simulink model "stereo_ibvs_core_backup_20260724_004703"  (R2025b)
settings: Solver=FixedStepDiscrete  StartTime=0.0  StopTime=inf  FixedStep=cfg.Ts  RelTol=1e-3
InitFcn:
  | cfgValid__=evalin('base','exist(''cfg'',''var'')==1 && isstruct(cfg) && all(isfield(cfg,{''Ts'',''robot'',''qInitial'',''zoomInitialSteps'',''cameraIntrinsicsStage1'',''rhoD'',''stereoBaseline'',''centerDesired'',''Kc'',''lambdaC'',''qMin'',''qMax'',''qLimitSoftMargin'',''qDotAlgorithmMax'',''stage1CalibrationReady''}))');if ~cfgValid__,modelFile__=get_param(bdroot,'FileName');modelDir__=fileparts(modelFile__);config1__=fullfile(modelDir__,'stereo_ibvs_config.m');config2__=fullfile(fileparts(modelDir__),'config','stereo_ibvs_config.m');if isfile(config1__),run(config1__);elseif isfile(config2__),run(config2__);else,error('StereoIBVS:ConfigNotFound','找不到stereo_ibvs_config.m。');end;end;clear cfgValid__ modelFile__ modelDir__ config1__ config2__
undefined symbols (not defined in the file): cfg, cfg_baseline, cfg_ekfCovarianceJitter, cfg_ekfInitializationMode, cfg_ekfP0, cfg_ekfRequireNewMeasurement, cfg_ekfSConditionMin, cfg_ekfX0, cfg_focalLength0Mm, cfg_fr3Axis, cfg_fr3Joint8OriginRPY, cfg_fr3Joint8OriginXYZ, cfg_fr3OriginRPY, cfg_fr3OriginXYZ, cfg_numericalEpsilon, cfg_pixelNoiseStd, cfg_q0, cfg_rhoMax, cfg_rhoMin, cfg_sigmaJerk, cfg_T_CL_CR, cfg_T_link8_CL, cfg_T_W_B, cfg_Ts, cfg_visibilityZMin
(part 2 of 4)

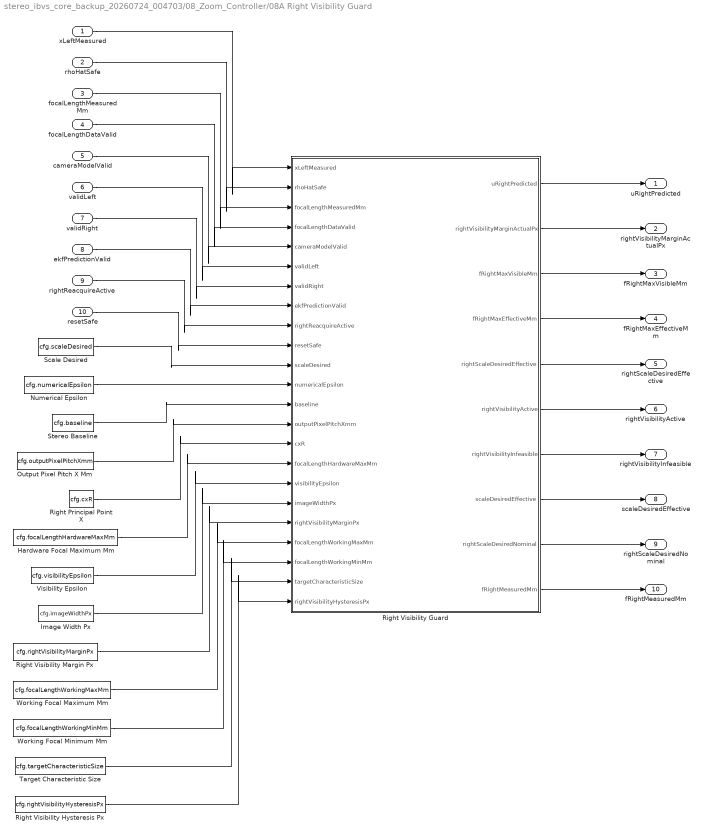
== system stereo_ibvs_core_backup_20260724_004703/08_Zoom_Controller/08A Right Visibility Guard ==
  xLeftMeasured : Inport  OutDataTypeStr=double  PortDimensions=1
  rhoHatSafe : Inport  Port=2  OutDataTypeStr=double  PortDimensions=1
  focalLengthMeasuredMm : Inport  Port=3  OutDataTypeStr=double  PortDimensions=[2 1]
  focalLengthDataValid : Inport  Port=4  OutDataTypeStr=double  PortDimensions=1
  cameraModelValid : Inport  Port=5  OutDataTypeStr=double  PortDimensions=1
  validLeft : Inport  Port=6  OutDataTypeStr=double  PortDimensions=1
  validRight : Inport  Port=7  OutDataTypeStr=double  PortDimensions=1
  ekfPredictionValid : Inport  Port=8  OutDataTypeStr=double  PortDimensions=1
  rightReacquireActive : Inport  Port=9  OutDataTypeStr=double  PortDimensions=1
  resetSafe : Inport  Port=10  OutDataTypeStr=double  PortDimensions=1
  Hardware Focal Maximum Mm : Constant  Value=cfg.focalLengthHardwareMaxMm  OutDataTypeStr=double  SampleTime=-1
  Image Width Px : Constant  Value=cfg.imageWidthPx  OutDataTypeStr=double  SampleTime=-1
  Numerical Epsilon : Constant  Value=cfg.numericalEpsilon  OutDataTypeStr=double  SampleTime=-1
  Output Pixel Pitch X Mm : Constant  Value=cfg.outputPixelPitchXmm  OutDataTypeStr=double  SampleTime=-1
  Right Principal Point X : Constant  Value=cfg.cxR  OutDataTypeStr=double  SampleTime=-1
  Right Visibility Guard : MATLAB Function  TreatAsAtomicUnit=on
  Right Visibility Hysteresis Px : Constant  Value=cfg.rightVisibilityHysteresisPx  OutDataTypeStr=double  SampleTime=-1
  Right Visibility Margin Px : Constant  Value=cfg.rightVisibilityMarginPx  OutDataTypeStr=double  SampleTime=-1
  Scale Desired : Constant  Value=cfg.scaleDesired  OutDataTypeStr=double  SampleTime=-1
  Stereo Baseline : Constant  Value=cfg.baseline  OutDataTypeStr=double  SampleTime=-1
  Target Characteristic Size : Constant  Value=cfg.targetCharacteristicSize  OutDataTypeStr=double  SampleTime=-1
  Visibility Epsilon : Constant  Value=cfg.visibilityEpsilon  OutDataTypeStr=double  SampleTime=-1
  Working Focal Maximum Mm : Constant  Value=cfg.focalLengthWorkingMaxMm  OutDataTypeStr=double  SampleTime=-1
  Working Focal Minimum Mm : Constant  Value=cfg.focalLengthWorkingMinMm  OutDataTypeStr=double  SampleTime=-1
  uRightPredicted : Outport  PortDimensions=1
  rightVisibilityMarginActualPx : Outport  Port=2  PortDimensions=1
  fRightMaxVisibleMm : Outport  Port=3  PortDimensions=1
  fRightMaxEffectiveMm : Outport  Port=4  PortDimensions=1
  rightScaleDesiredEffective : Outport  Port=5  PortDimensions=1
  rightVisibilityActive : Outport  Port=6  PortDimensions=1
  rightVisibilityInfeasible : Outport  Port=7  PortDimensions=1
  scaleDesiredEffective : Outport  Port=8  PortDimensions=[2 1]
  rightScaleDesiredNominal : Outport  Port=9  PortDimensions=1
  fRightMeasuredMm : Outport  Port=10  PortDimensions=1
  wires:
  Right Visibility Guard/9(rightScaleDesiredNominal) -> rightScaleDesiredNominal/1
  Right Visibility Guard/7(rightVisibilityInfeasible) -> rightVisibilityInfeasible/1
  Scale Desired/1 -> Right Visibility Guard/11(scaleDesired)
  Right Visibility Guard/6(rightVisibilityActive) -> rightVisibilityActive/1
  rightReacquireActive/1 -> Right Visibility Guard/9(rightReacquireActive)
  ekfPredictionValid/1 -> Right Visibility Guard/8(ekfPredictionValid)
  resetSafe/1 -> Right Visibility Guard/10(resetSafe)
  Stereo Baseline/1 -> Right Visibility Guard/13(baseline)
  validLeft/1 -> Right Visibility Guard/6(validLeft)
  Working Focal Minimum Mm/1 -> Right Visibility Guard/21(focalLengthWorkingMinMm)
  rhoHatSafe/1 -> Right Visibility Guard/2(rhoHatSafe)
  focalLengthDataValid/1 -> Right Visibility Guard/4(focalLengthDataValid)
  cameraModelValid/1 -> Right Visibility Guard/5(cameraModelValid)
  validRight/1 -> Right Visibility Guard/7(validRight)
  Right Visibility Guard/8(scaleDesiredEffective) -> scaleDesiredEffective/1
  Hardware Focal Maximum Mm/1 -> Right Visibility Guard/16(focalLengthHardwareMaxMm)
  Image Width Px/1 -> Right Visibility Guard/18(imageWidthPx)
  Output Pixel Pitch X Mm/1 -> Right Visibility Guard/14(outputPixelPitchXmm)
  Right Visibility Guard/10(fRightMeasuredMm) -> fRightMeasuredMm/1
  Right Principal Point X/1 -> Right Visibility Guard/15(cxR)
  Target Characteristic Size/1 -> Right Visibility Guard/22(targetCharacteristicSize)
  Visibility Epsilon/1 -> Right Visibility Guard/17(visibilityEpsilon)
  Right Visibility Guard/2(rightVisibilityMarginActualPx) -> rightVisibilityMarginActualPx/1
  Right Visibility Guard/4(fRightMaxEffectiveMm) -> fRightMaxEffectiveMm/1
  Numerical Epsilon/1 -> Right Visibility Guard/12(numericalEpsilon)
  Right Visibility Guard/3(fRightMaxVisibleMm) -> fRightMaxVisibleMm/1
  Working Focal Maximum Mm/1 -> Right Visibility Guard/20(focalLengthWorkingMaxMm)
  Right Visibility Guard/1(uRightPredicted) -> uRightPredicted/1
  Right Visibility Margin Px/1 -> Right Visibility Guard/19(rightVisibilityMarginPx)
  Right Visibility Hysteresis Px/1 -> Right Visibility Guard/23(rightVisibilityHysteresisPx)
  focalLengthMeasuredMm/1 -> Right Visibility Guard/3(focalLengthMeasuredMm)
  xLeftMeasured/1 -> Right Visibility Guard/1(xLeftMeasured)
  Right Visibility Guard/5(rightScaleDesiredEffective) -> rightScaleDesiredEffective/1

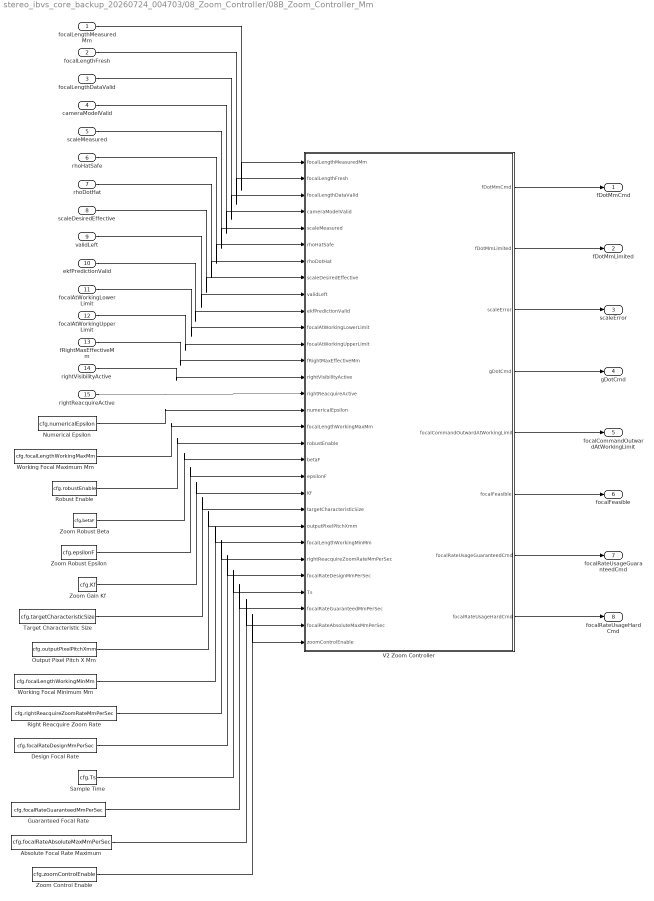
== system stereo_ibvs_core_backup_20260724_004703/08_Zoom_Controller/08B_Zoom_Controller_Mm ==
  focalLengthMeasuredMm : Inport  OutDataTypeStr=double  PortDimensions=[2 1]
  focalLengthFresh : Inport  Port=2  OutDataTypeStr=double  PortDimensions=1
  focalLengthDataValid : Inport  Port=3  OutDataTypeStr=double  PortDimensions=1
  cameraModelValid : Inport  Port=4  OutDataTypeStr=double  PortDimensions=1
  scaleMeasured : Inport  Port=5  OutDataTypeStr=double  PortDimensions=[2 1]
  rhoHatSafe : Inport  Port=6  OutDataTypeStr=double  PortDimensions=1
  rhoDotHat : Inport  Port=7  OutDataTypeStr=double  PortDimensions=[2 1]
  scaleDesiredEffective : Inport  Port=8  OutDataTypeStr=double  PortDimensions=[2 1]
  validLeft : Inport  Port=9  OutDataTypeStr=double  PortDimensions=1
  ekfPredictionValid : Inport  Port=10  OutDataTypeStr=double  PortDimensions=1
  focalAtWorkingLowerLimit : Inport  Port=11  OutDataTypeStr=double  PortDimensions=[2 1]
  focalAtWorkingUpperLimit : Inport  Port=12  OutDataTypeStr=double  PortDimensions=[2 1]
  fRightMaxEffectiveMm : Inport  Port=13  OutDataTypeStr=double  PortDimensions=1
  rightVisibilityActive : Inport  Port=14  OutDataTypeStr=double  PortDimensions=1
  rightReacquireActive : Inport  Port=15  OutDataTypeStr=double  PortDimensions=1
  Absolute Focal Rate Maximum : Constant  Value=cfg.focalRateAbsoluteMaxMmPerSec  OutDataTypeStr=double  SampleTime=-1
  Design Focal Rate : Constant  Value=cfg.focalRateDesignMmPerSec  OutDataTypeStr=double  SampleTime=-1
  Guaranteed Focal Rate : Constant  Value=cfg.focalRateGuaranteedMmPerSec  OutDataTypeStr=double  SampleTime=-1
  Numerical Epsilon : Constant  Value=cfg.numericalEpsilon  OutDataTypeStr=double  SampleTime=-1
  Output Pixel Pitch X Mm : Constant  Value=cfg.outputPixelPitchXmm  OutDataTypeStr=double  SampleTime=-1
  Right Reacquire Zoom Rate : Constant  Value=cfg.rightReacquireZoomRateMmPerSec  OutDataTypeStr=double  SampleTime=-1
  Robust Enable : Constant  Value=cfg.robustEnable  OutDataTypeStr=double  SampleTime=-1
  Sample Time : Constant  Value=cfg.Ts  OutDataTypeStr=double  SampleTime=-1
  Target Characteristic Size : Constant  Value=cfg.targetCharacteristicSize  OutDataTypeStr=double  SampleTime=-1
  V2 Zoom Controller : MATLAB Function  TreatAsAtomicUnit=on
  Working Focal Maximum Mm : Constant  Value=cfg.focalLengthWorkingMaxMm  OutDataTypeStr=double  SampleTime=-1
  Working Focal Minimum Mm : Constant  Value=cfg.focalLengthWorkingMinMm  OutDataTypeStr=double  SampleTime=-1
  Zoom Control Enable : Constant  Value=cfg.zoomControlEnable  OutDataTypeStr=double  SampleTime=-1
  Zoom Gain Kf : Constant  Value=cfg.Kf  OutDataTypeStr=double  SampleTime=-1
  Zoom Robust Beta : Constant  Value=cfg.betaF  OutDataTypeStr=double  SampleTime=-1
  Zoom Robust Epsilon : Constant  Value=cfg.epsilonF  OutDataTypeStr=double  SampleTime=-1
  fDotMmCmd : Outport  PortDimensions=[2 1]
  fDotMmLimited : Outport  Port=2  PortDimensions=[2 1]
  scaleError : Outport  Port=3  PortDimensions=[2 1]
  gDotCmd : Outport  Port=4  PortDimensions=[2 1]
  focalCommandOutwardAtWorkingLimit : Outport  Port=5  PortDimensions=[2 1]
  focalFeasible : Outport  Port=6  PortDimensions=[2 1]
  focalRateUsageGuaranteedCmd : Outport  Port=7  PortDimensions=[2 1]
  focalRateUsageHardCmd : Outport  Port=8  PortDimensions=[2 1]
  wires:
  V2 Zoom Controller/6(focalFeasible) -> focalFeasible/1
  V2 Zoom Controller/4(gDotCmd) -> gDotCmd/1
  V2 Zoom Controller/3(scaleError) -> scaleError/1
  V2 Zoom Controller/1(fDotMmCmd) -> fDotMmCmd/1
  Zoom Control Enable/1 -> V2 Zoom Controller/30(zoomControlEnable)
  V2 Zoom Controller/8(focalRateUsageHardCmd) -> focalRateUsageHardCmd/1
  focalAtWorkingUpperLimit/1 -> V2 Zoom Controller/12(focalAtWorkingUpperLimit)
  ekfPredictionValid/1 -> V2 Zoom Controller/10(ekfPredictionValid)
  V2 Zoom Controller/5(focalCommandOutwardAtWorkingLimit) -> focalCommandOutwardAtWorkingLimit/1
  focalAtWorkingLowerLimit/1 -> V2 Zoom Controller/11(focalAtWorkingLowerLimit)
  Zoom Gain Kf/1 -> V2 Zoom Controller/21(Kf)
  scaleMeasured/1 -> V2 Zoom Controller/5(scaleMeasured)
  rhoDotHat/1 -> V2 Zoom Controller/7(rhoDotHat)
  rhoHatSafe/1 -> V2 Zoom Controller/6(rhoHatSafe)
  V2 Zoom Controller/2(fDotMmLimited) -> fDotMmLimited/1
  Working Focal Maximum Mm/1 -> V2 Zoom Controller/17(focalLengthWorkingMaxMm)
  focalLengthDataValid/1 -> V2 Zoom Controller/3(focalLengthDataValid)
  focalLengthFresh/1 -> V2 Zoom Controller/2(focalLengthFresh)
  fRightMaxEffectiveMm/1 -> V2 Zoom Controller/13(fRightMaxEffectiveMm)
  validLeft/1 -> V2 Zoom Controller/9(validLeft)
  Numerical Epsilon/1 -> V2 Zoom Controller/16(numericalEpsilon)
  focalLengthMeasuredMm/1 -> V2 Zoom Controller/1(focalLengthMeasuredMm)
  Working Focal Minimum Mm/1 -> V2 Zoom Controller/24(focalLengthWorkingMinMm)
  rightReacquireActive/1 -> V2 Zoom Controller/15(rightReacquireActive)
  Robust Enable/1 -> V2 Zoom Controller/18(robustEnable)
  Target Characteristic Size/1 -> V2 Zoom Controller/22(targetCharacteristicSize)
  rightVisibilityActive/1 -> V2 Zoom Controller/14(rightVisibilityActive)
  cameraModelValid/1 -> V2 Zoom Controller/4(cameraModelValid)
  Zoom Robust Beta/1 -> V2 Zoom Controller/19(betaF)
  scaleDesiredEffective/1 -> V2 Zoom Controller/8(scaleDesiredEffective)
  Zoom Robust Epsilon/1 -> V2 Zoom Controller/20(epsilonF)
  Output Pixel Pitch X Mm/1 -> V2 Zoom Controller/23(outputPixelPitchXmm)
  Design Focal Rate/1 -> V2 Zoom Controller/26(focalRateDesignMmPerSec)
  Sample Time/1 -> V2 Zoom Controller/27(Ts)
  Guaranteed Focal Rate/1 -> V2 Zoom Controller/28(focalRateGuaranteedMmPerSec)
  V2 Zoom Controller/7(focalRateUsageGuaranteedCmd) -> focalRateUsageGuaranteedCmd/1
  Right Reacquire Zoom Rate/1 -> V2 Zoom Controller/25(rightReacquireZoomRateMmPerSec)
  Absolute Focal Rate Maximum/1 -> V2 Zoom Controller/29(focalRateAbsoluteMaxMmPerSec)

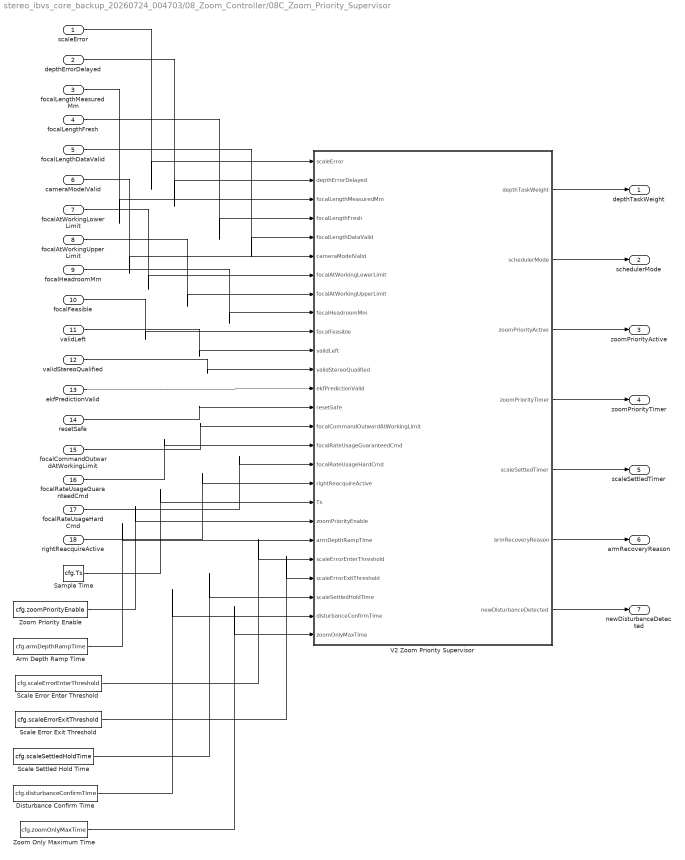
== system stereo_ibvs_core_backup_20260724_004703/08_Zoom_Controller/08C_Zoom_Priority_Supervisor ==
  scaleError : Inport  OutDataTypeStr=double  PortDimensions=[2 1]
  depthErrorDelayed : Inport  Port=2  OutDataTypeStr=double  PortDimensions=1
  focalLengthMeasuredMm : Inport  Port=3  OutDataTypeStr=double  PortDimensions=[2 1]
  focalLengthFresh : Inport  Port=4  OutDataTypeStr=double  PortDimensions=1
  focalLengthDataValid : Inport  Port=5  OutDataTypeStr=double  PortDimensions=1
  cameraModelValid : Inport  Port=6  OutDataTypeStr=double  PortDimensions=1
  focalAtWorkingLowerLimit : Inport  Port=7  OutDataTypeStr=double  PortDimensions=[2 1]
  focalAtWorkingUpperLimit : Inport  Port=8  OutDataTypeStr=double  PortDimensions=[2 1]
  focalHeadroomMm : Inport  Port=9  OutDataTypeStr=double  PortDimensions=[2 1]
  focalFeasible : Inport  Port=10  OutDataTypeStr=double  PortDimensions=[2 1]
  validLeft : Inport  Port=11  OutDataTypeStr=double  PortDimensions=1
  validStereoQualified : Inport  Port=12  OutDataTypeStr=double  PortDimensions=1
  ekfPredictionValid : Inport  Port=13  OutDataTypeStr=double  PortDimensions=1
  resetSafe : Inport  Port=14  OutDataTypeStr=double  PortDimensions=1
  focalCommandOutwardAtWorkingLimit : Inport  Port=15  OutDataTypeStr=double  PortDimensions=[2 1]
  focalRateUsageGuaranteedCmd : Inport  Port=16  OutDataTypeStr=double  PortDimensions=[2 1]
  focalRateUsageHardCmd : Inport  Port=17  OutDataTypeStr=double  PortDimensions=[2 1]
  rightReacquireActive : Inport  Port=18  OutDataTypeStr=double  PortDimensions=1
  Arm Depth Ramp Time : Constant  Value=cfg.armDepthRampTime  OutDataTypeStr=double  SampleTime=-1
  Disturbance Confirm Time : Constant  Value=cfg.disturbanceConfirmTime  OutDataTypeStr=double  SampleTime=-1
  Sample Time : Constant  Value=cfg.Ts  OutDataTypeStr=double  SampleTime=-1
  Scale Error Enter Threshold : Constant  Value=cfg.scaleErrorEnterThreshold  OutDataTypeStr=double  SampleTime=-1
  Scale Error Exit Threshold : Constant  Value=cfg.scaleErrorExitThreshold  OutDataTypeStr=double  SampleTime=-1
  Scale Settled Hold Time : Constant  Value=cfg.scaleSettledHoldTime  OutDataTypeStr=double  SampleTime=-1
  V2 Zoom Priority Supervisor : MATLAB Function  TreatAsAtomicUnit=on
  Zoom Only Maximum Time : Constant  Value=cfg.zoomOnlyMaxTime  OutDataTypeStr=double  SampleTime=-1
  Zoom Priority Enable : Constant  Value=cfg.zoomPriorityEnable  OutDataTypeStr=double  SampleTime=-1
  depthTaskWeight : Outport  PortDimensions=1
  schedulerMode : Outport  Port=2  PortDimensions=1
  zoomPriorityActive : Outport  Port=3  PortDimensions=1
  zoomPriorityTimer : Outport  Port=4  PortDimensions=1
  scaleSettledTimer : Outport  Port=5  PortDimensions=1
  armRecoveryReason : Outport  Port=6  PortDimensions=1
  newDisturbanceDetected : Outport  Port=7  PortDimensions=1
  wires:
  V2 Zoom Priority Supervisor/7(newDisturbanceDetected) -> newDisturbanceDetected/1
  V2 Zoom Priority Supervisor/6(armRecoveryReason) -> armRecoveryReason/1
  V2 Zoom Priority Supervisor/4(zoomPriorityTimer) -> zoomPriorityTimer/1
  validLeft/1 -> V2 Zoom Priority Supervisor/11(validLeft)
  focalFeasible/1 -> V2 Zoom Priority Supervisor/10(focalFeasible)
  ekfPredictionValid/1 -> V2 Zoom Priority Supervisor/13(ekfPredictionValid)
  focalAtWorkingLowerLimit/1 -> V2 Zoom Priority Supervisor/7(focalAtWorkingLowerLimit)
  Zoom Only Maximum Time/1 -> V2 Zoom Priority Supervisor/26(zoomOnlyMaxTime)
  cameraModelValid/1 -> V2 Zoom Priority Supervisor/6(cameraModelValid)
  scaleError/1 -> V2 Zoom Priority Supervisor/1(scaleError)
  focalLengthDataValid/1 -> V2 Zoom Priority Supervisor/5(focalLengthDataValid)
  focalRateUsageHardCmd/1 -> V2 Zoom Priority Supervisor/17(focalRateUsageHardCmd)
  V2 Zoom Priority Supervisor/5(scaleSettledTimer) -> scaleSettledTimer/1
  V2 Zoom Priority Supervisor/2(schedulerMode) -> schedulerMode/1
  focalLengthFresh/1 -> V2 Zoom Priority Supervisor/4(focalLengthFresh)
  Scale Settled Hold Time/1 -> V2 Zoom Priority Supervisor/24(scaleSettledHoldTime)
  V2 Zoom Priority Supervisor/1(depthTaskWeight) -> depthTaskWeight/1
  resetSafe/1 -> V2 Zoom Priority Supervisor/14(resetSafe)
  focalRateUsageGuaranteedCmd/1 -> V2 Zoom Priority Supervisor/16(focalRateUsageGuaranteedCmd)
  rightReacquireActive/1 -> V2 Zoom Priority Supervisor/18(rightReacquireActive)
  Sample Time/1 -> V2 Zoom Priority Supervisor/19(Ts)
  focalAtWorkingUpperLimit/1 -> V2 Zoom Priority Supervisor/8(focalAtWorkingUpperLimit)
  focalCommandOutwardAtWorkingLimit/1 -> V2 Zoom Priority Supervisor/15(focalCommandOutwardAtWorkingLimit)
  Zoom Priority Enable/1 -> V2 Zoom Priority Supervisor/20(zoomPriorityEnable)
  depthErrorDelayed/1 -> V2 Zoom Priority Supervisor/2(depthErrorDelayed)
  Arm Depth Ramp Time/1 -> V2 Zoom Priority Supervisor/21(armDepthRampTime)
  Scale Error Enter Threshold/1 -> V2 Zoom Priority Supervisor/22(scaleErrorEnterThreshold)
  Scale Error Exit Threshold/1 -> V2 Zoom Priority Supervisor/23(scaleErrorExitThreshold)
  validStereoQualified/1 -> V2 Zoom Priority Supervisor/12(validStereoQualified)
  focalHeadroomMm/1 -> V2 Zoom Priority Supervisor/9(focalHeadroomMm)
  Disturbance Confirm Time/1 -> V2 Zoom Priority Supervisor/25(disturbanceConfirmTime)
  focalLengthMeasuredMm/1 -> V2 Zoom Priority Supervisor/3(focalLengthMeasuredMm)
  V2 Zoom Priority Supervisor/3(zoomPriorityActive) -> zoomPriorityActive/1

== matlab function stereo_ibvs_core_backup_20260724_004703/02_Camera_and_Zoom_Model/V2_Camera_and_Zoom_Model ==
  data: focalLengthMeasuredMmRaw input; focalLengthMeasuredMm output; focalLengthIsNew input; resetSafe input; cfg_focalLengthHardwareMinMm input; cfg_focalLengthHardwareMaxMm input; cfg_focalLengthWorkingMinMm input; cfg_focalLengthWorkingMaxMm input; cfg_outputPixelPitchXmm input; cfg_outputPixelPitchYmm input; cfg_focalLengthTimeoutFrames input; cfg_numericalEpsilon input; fxMeasuredPx output; fyMeasuredPx output; focalLengthFresh output; focalLengthDataValid output; focalAtWorkingLowerLimit output; focalAtWorkingUpperLimit output; focalAtHardwareLowerLimit output; focalAtHardwareUpperLimit output; focalOutsideWorkingRange output; focalHardwareLimitViolation output; focalRangeUsage output; focalHeadroomMm output; cameraModelValid output
function [ ...
    focalLengthMeasuredMm, ...
    fxMeasuredPx, ...
    fyMeasuredPx, ...
    focalLengthFresh, ...
    focalLengthDataValid, ...
    focalAtWorkingLowerLimit, ...
    focalAtWorkingUpperLimit, ...
    focalAtHardwareLowerLimit, ...
    focalAtHardwareUpperLimit, ...
    focalOutsideWorkingRange, ...
    focalHardwareLimitViolation, ...
    focalRangeUsage, ...
    focalHeadroomMm, ...
    cameraModelValid] = fcn( ...
    focalLengthMeasuredMmRaw, ...
    focalLengthIsNew, ...
    resetSafe, ...
    cfg_focalLengthHardwareMinMm, ...
    cfg_focalLengthHardwareMaxMm, ...
    cfg_focalLengthWorkingMinMm, ...
    cfg_focalLengthWorkingMaxMm, ...
    cfg_outputPixelPitchXmm, ...
    cfg_outputPixelPitchYmm, ...
    cfg_focalLengthTimeoutFrames, ...
    cfg_numericalEpsilon)
%#codegen
% V2 Camera and Zoom Model
%
% 焦距反馈：
% [fL_mm; fR_mm]
%
% 超时后保持最后一次有效焦距，但 focalLengthFresh = false。
% 08模块应在 focalLengthFresh = false 时停止Zoom命令。

%% 固定尺寸输入
focalRaw = reshape(focalLengthMeasuredMmRaw,2,1);

hardwareMin = reshape( ...
    cfg_focalLengthHardwareMinMm,2,1);

hardwareMax = reshape( ...
    cfg_focalLengthHardwareMaxMm,2,1);

workingMin = reshape( ...
    cfg_focalLengthWorkingMinMm,2,1);

workingMax = reshape( ...
    cfg_focalLengthWorkingMaxMm,2,1);

%% 持久状态
persistent lastValidFocalLengthMm
persistent focalLengthReceivedOnce
persistent framesSinceLastValidMessage

if isempty(lastValidFocalLengthMm)
    lastValidFocalLengthMm = zeros(2,1);
    focalLengthReceivedOnce = false;
    framesSinceLastValidMessage = ...
        double(cfg_focalLengthTimeoutFrames);
end

%% 固定尺寸输出
focalLengthMeasuredMm = zeros(2,1);
fxMeasuredPx = zeros(2,1);
fyMeasuredPx = zeros(2,1);

focalLengthFresh = false;
focalLengthDataValid = false;

focalAtWorkingLowerLimit = false(2,1);
focalAtWorkingUpperLimit = false(2,1);
focalAtHardwareLowerLimit = false(2,1);
focalAtHardwareUpperLimit = false(2,1);

focalOutsideWorkingRange = false(2,1);
focalHardwareLimitViolation = false(2,1);

focalRangeUsage = zeros(2,1);
focalHeadroomMm = zeros(2,1);

cameraModelValid = false;

%% 配置检查
numericalConfigurationValid = ...
    isfinite(cfg_numericalEpsilon) && ...
    cfg_numericalEpsilon > 0;

hardwareRangeValid = ...
    all(isfinite(hardwareMin)) && ...
    all(isfinite(hardwareMax)) && ...
    all(hardwareMax > hardwareMin);

workingRangeValid = ...
    all(isfinite(workingMin)) && ...
    all(isfinite(workingMax)) && ...
    all(workingMax > workingMin) && ...
    all(workingMin >= hardwareMin) && ...
    all(workingMax <= hardwareMax);

pixelPitchValid = ...
    isfinite(cfg_outputPixelPitchXmm) && ...
    isfinite(cfg_outputPixelPitchYmm) && ...
    cfg_outputPixelPitchXmm > cfg_numericalEpsilon && ...
    cfg_outputPixelPitchYmm > cfg_numericalEpsilon;

timeoutConfigurationValid = ...
    isfinite(cfg_focalLengthTimeoutFrames) && ...
    cfg_focalLengthTimeoutFrames >= 1;

configurationValid = ...
    numericalConfigurationValid && ...
    hardwareRangeValid && ...
    workingRangeValid && ...
    pixelPitchValid && ...
    timeoutConfigurationValid;

%% 控制输入检查
controlSignalsFinite = ...
    isfinite(focalLengthIsNew) && ...
    isfinite(resetSafe);

%% 复位或更新焦距状态
if ~controlSignalsFinite || resetSafe > 0.5

    lastValidFocalLengthMm = zeros(2,1);
    focalLengthReceivedOnce = false;
    framesSinceLastValidMessage = ...
        double(cfg_focalLengthTimeoutFrames);

else

    rawFinite = all(isfinite(focalRaw));

    rawInsideHardwareRange = ...
        rawFinite && ...
        hardwareRangeValid && ...
        all(focalRaw >= hardwareMin) && ...
        all(focalRaw <= hardwareMax);

    newValidMessage = ...
        focalLengthIsNew > 0.5 && ...
        rawInsideHardwareRange && ...
        configurationValid;

    if newValidMessage

        lastValidFocalLengthMm = focalRaw;
        focalLengthReceivedOnce = true;
        framesSinceLastValidMessage = 0;

    elseif focalLengthReceivedOnce

        maximumCounterValue = ...
            double(cfg_focalLengthTimeoutFrames) + 1;

        framesSinceLastValidMessage = min( ...
            framesSinceLastValidMessage + 1, ...
            maximumCounterValue);
    end
end

%% 输出最近一次有效焦距
if focalLengthReceivedOnce
    focalLengthMeasuredMm = ...
        lastValidFocalLengthMm;
end

%% 焦距新鲜度
focalLengthFresh = ...
    focalLengthReceivedOnce && ...
    framesSinceLastValidMessage < ...
        double(cfg_focalLengthTimeoutFrames);

%% 保存焦距有效性
if focalLengthReceivedOnce && hardwareRangeValid

    focalLengthDataValid = ...
        all(isfinite(focalLengthMeasuredMm)) && ...
        all(focalLengthMeasuredMm >= hardwareMin) && ...
        all(focalLengthMeasuredMm <= hardwareMax);
end

%% 焦距范围状态
if focalLengthReceivedOnce && configurationValid

    focalAtWorkingLowerLimit = ...
        focalLengthMeasuredMm <= workingMin;

    focalAtWorkingUpperLimit = ...
        focalLengthMeasuredMm >= workingMax;

    focalAtHardwareLowerLimit = ...
        focalLengthMeasuredMm <= hardwareMin;

    focalAtHardwareUpperLimit = ...
        focalLengthMeasuredMm >= hardwareMax;

    focalOutsideWorkingRange = ...
        focalLengthMeasuredMm < workingMin | ...
        focalLengthMeasuredMm > workingMax;

    focalHardwareLimitViolation = ...
        focalLengthMeasuredMm < hardwareMin | ...
        focalLengthMeasuredMm > hardwareMax;

    workingRangeWidth = ...
        workingMax - workingMin;

    focalRangeUsage = ...
        (focalLengthMeasuredMm-workingMin) ./ ...
        workingRangeWidth;

    focalRangeUsage = min( ...
        max(focalRangeUsage,zeros(2,1)), ...
        ones(2,1));

    lowerHeadroomMm = ...
        focalLengthMeasuredMm-workingMin;

    upperHeadroomMm = ...
        workingMax-focalLengthMeasuredMm;

    focalHeadroomMm = max( ...
        min(lowerHeadroomMm,upperHeadroomMm), ...
        zeros(2,1));
end

%% 焦距mm转换为像素焦距
cameraModelValid = ...
    configurationValid && ...
    focalLengthDataValid && ...
    ~any(focalHardwareLimitViolation);

if cameraModelValid

    fxMeasuredPx = ...
        focalLengthMeasuredMm ./ ...
        cfg_outputPixelPitchXmm;

    fyMeasuredPx = ...
        focalLengthMeasuredMm ./ ...
        cfg_outputPixelPitchYmm;
end

%% 最终有限值保护
outputFinite = ...
    all(isfinite(focalLengthMeasuredMm)) && ...
    all(isfinite(fxMeasuredPx)) && ...
    all(isfinite(fyMeasuredPx)) && ...
    all(isfinite(focalRangeUsage)) && ...
    all(isfinite(focalHeadroomMm));

if ~outputFinite

    focalLengthMeasuredMm = zeros(2,1);
    fxMeasuredPx = zeros(2,1);
    fyMeasuredPx = zeros(2,1);

    focalLengthFresh = false;
    focalLengthDataValid = false;

    focalAtWorkingLowerLimit = false(2,1);
    focalAtWorkingUpperLimit = false(2,1);
    focalAtHardwareLowerLimit = false(2,1);
    focalAtHardwareUpperLimit = false(2,1);

    focalOutsideWorkingRange = false(2,1);
    focalHardwareLimitViolation = false(2,1);

    focalRangeUsage = zeros(2,1);
    focalHeadroomMm = zeros(2,1);

    cameraModelValid = false;
end
end

== matlab function stereo_ibvs_core_backup_20260724_004703/07_Arm_Priority_Controller/Final Arm Priority Controller ==
  data: q input; qDotCmd output; cLMeasured input; rhoHatL input; vHatLeft input; JL input; cLd input; rhoD input; validLeft input; ekfPredictionValid input; centerEnable input; depthEnable input; armEnable input; depthTaskWeight input; cfg_numericalEpsilon input; cfg_robustEnable input; cfg_betaC input; cfg_epsilonC input; cfg_Kc input; cfg_lambdaC input; cfg_betaRho input; cfg_epsilonRho input; cfg_kRho input; cfg_lambdaRho input; cfg_nullspaceEnable input; cfg_kNull input; cfg_qMid input; cfg_leftOnlyCenterControlEnable input; centerError output; depthError output; rcondJc output; rcondArho output; qDotCenter output; qDotDepthRaw output; qDotDepthWeighted output; qDotNullUsed output
function [qDotCmd,centerError,depthError,rcondJc,rcondArho,qDotCenter,qDotDepthRaw,qDotDepthWeighted,qDotNullUsed] = ...
    fcn(q,cLMeasured,rhoHatL,vHatLeft,JL,cLd,rhoD,validLeft,ekfPredictionValid,centerEnable,depthEnable,armEnable,depthTaskWeight, ...
    cfg_numericalEpsilon,cfg_robustEnable,cfg_betaC,cfg_epsilonC,cfg_Kc,cfg_lambdaC,cfg_betaRho,cfg_epsilonRho,cfg_kRho,cfg_lambdaRho,cfg_nullspaceEnable,cfg_kNull,cfg_qMid,cfg_leftOnlyCenterControlEnable)
%#codegen
% 代码作用：
% 左相机归一化中心为主任务，逆深度为次任务。
% 支持目标速度前馈、鲁棒项、阻尼伪逆和关节中位零空间任务。

qDotCmd = zeros(7,1);
centerError = zeros(2,1);
depthError = 0;
rcondJc = 0;
rcondArho = 0;
qDotCenter = zeros(7,1);
qDotDepthRaw = zeros(7,1);
qDotDepthWeighted = zeros(7,1);
qDotNullUsed = zeros(7,1);

x = cLMeasured(1);
y = cLMeasured(2);
rho = rhoD;
vFeed = zeros(3,1);

if ekfPredictionValid > 0.5 && ...
        isfinite(rhoHatL) && rhoHatL > 0 && ...
        all(isfinite(vHatLeft))
    rho = max(rhoHatL,cfg_numericalEpsilon);
    vFeed = vHatLeft;
end

centerError = [x;y] - cLd;
depthError = rho - rhoD;

Lc = [
    -rho, 0, x*rho, x*y, -(1+x*x), y
    0, -rho, y*rho, 1+y*y, -x*y, -x
];

Hc = rho*[1 0 -x;0 1 -y];
bhatC = Hc*vFeed;
Jc = Lc*JL;

rc = zeros(2,1);
if cfg_robustEnable > 0.5
    rc = cfg_betaC*centerError / ...
        (sqrt(centerError'*centerError)+cfg_epsilonC);
end

nuC = -cfg_Kc*centerError - bhatC - rc;
Gc = Jc*Jc' + cfg_lambdaC^2*eye(2);
JcSharp = Jc'/Gc;
qC = JcSharp*nuC;
Nc = eye(7)-JcSharp*Jc;
rcondJc = det(Gc) / ...
    (trace(Gc)*trace(Gc)+cfg_numericalEpsilon);
qDotCenter = qC;

Lrho = [0 0 rho*rho rho*y -rho*x 0];
Hrho = [0 0 -rho*rho];
Jrho = Lrho*JL;
bhatRho = Hrho*vFeed;

rr = 0;
if cfg_robustEnable > 0.5
    rr = cfg_betaRho*depthError / ...
        (abs(depthError)+cfg_epsilonRho);
end

nuRho = -cfg_kRho*depthError-bhatRho-rr;
A = Jrho*Nc;
denom = A*A'+cfg_lambdaRho^2;
rcondArho = denom/(1+denom);

w = min(max(depthTaskWeight,0),1) * ...
    double(ekfPredictionValid > 0.5);
qDotDepthRaw = Nc*A'*((nuRho-Jrho*qC)/denom);
qDotDepthWeighted = w*qDotDepthRaw;

qDot0 = zeros(7,1);
if cfg_nullspaceEnable > 0.5
    qDot0 = -cfg_kNull*(q-cfg_qMid);
end

ArhoDagger = A'/denom;
NcRho = Nc*(eye(7)-ArhoDagger*A);
Nnull = (1-w)*Nc+w*NcRho;
qDotNullUsed = Nnull*qDot0;

if centerEnable > 0.5
    qDotCmd = qDotCenter+qDotNullUsed;
end

if centerEnable > 0.5 && depthEnable > 0.5
    qDotCmd = qDotCenter+qDotDepthWeighted+qDotNullUsed;
end

if centerEnable <= 0.5 && depthEnable > 0.5
    d = Jrho*Jrho'+cfg_lambdaRho^2;
    qDotDepthRaw = Jrho'*(nuRho/d);
    qDotDepthWeighted = w*qDotDepthRaw;
    qDotCenter = zeros(7,1);
    qDotNullUsed = zeros(7,1);
    qDotCmd = qDotDepthWeighted;
end

centerAllowed = validLeft > 0.5 && ...
    cfg_leftOnlyCenterControlEnable > 0.5;

if ~centerAllowed || armEnable <= 0.5
    qDotCmd = zeros(7,1);
    qDotCenter = zeros(7,1);
    qDotDepthWeighted = zeros(7,1);
    qDotNullUsed = zeros(7,1);
end

if any(~isfinite(qDotCmd))
    qDotCmd = zeros(7,1);
end
end

== matlab function stereo_ibvs_core_backup_20260724_004703/10_Diagnostics/V2_Output_and_Diagnostics ==
  data: qDotApplied input; jointVelocityCmd output; fDotMmApplied input; inputDataValid input; cameraModelValid input; focalLengthFresh input; kinematicsValid input; validLeft input; validRight input; validStereoQualified input; ekfPredictionValid input; ekfMeasurementUpdated input; depthTaskWeight input; schedulerMode input; safetyValid input; controllerEnableSafe input; focalRateCmdMmPerSec output; controllerStatus output
function [ ...
    jointVelocityCmd, ...
    focalRateCmdMmPerSec, ...
    controllerStatus] = fcn( ...
    qDotApplied, ...
    fDotMmApplied, ...
    inputDataValid, ...
    cameraModelValid, ...
    focalLengthFresh, ...
    kinematicsValid, ...
    validLeft, ...
    validRight, ...
    validStereoQualified, ...
    ekfPredictionValid, ...
    ekfMeasurementUpdated, ...
    depthTaskWeight, ...
    schedulerMode, ...
    safetyValid, ...
    controllerEnableSafe)
%#codegen
% V2 Output and Diagnostics
%
% jointVelocityCmd:
% [qDot1; ...; qDot7]，单位 rad/s
%
% focalRateCmdMmPerSec:
% [fDotLeft; fDotRight]，单位 mm/s
%
% 不再进行焦距速度到step/s的转换。

%% 固定尺寸输出
jointVelocityCmd = zeros(7,1);
focalRateCmdMmPerSec = zeros(2,1);
controllerStatus = zeros(13,1);

%% 固定尺寸输入
qDot = reshape(qDotApplied,7,1);
fDotMm = reshape(fDotMmApplied,2,1);

%% 状态信号整理
statusInputDataValid = double( ...
    isfinite(inputDataValid) && ...
    inputDataValid > 0.5);

statusCameraModelValid = double( ...
    isfinite(cameraModelValid) && ...
    cameraModelValid > 0.5);

statusFocalLengthFresh = double( ...
    isfinite(focalLengthFresh) && ...
    focalLengthFresh > 0.5);

statusKinematicsValid = double( ...
    isfinite(kinematicsValid) && ...
    kinematicsValid > 0.5);

statusValidLeft = double( ...
    isfinite(validLeft) && ...
    validLeft > 0.5);

statusValidRight = double( ...
    isfinite(validRight) && ...
    validRight > 0.5);

statusValidStereoQualified = double( ...
    isfinite(validStereoQualified) && ...
    validStereoQualified > 0.5);

statusEkfPredictionValid = double( ...
    isfinite(ekfPredictionValid) && ...
    ekfPredictionValid > 0.5);

statusEkfMeasurementUpdated = double( ...
    isfinite(ekfMeasurementUpdated) && ...
    ekfMeasurementUpdated > 0.5);

if isfinite(depthTaskWeight)
    statusDepthTaskWeight = ...
        min(max(depthTaskWeight,0),1);
else
    statusDepthTaskWeight = 0;
end

if isfinite(schedulerMode)
    statusSchedulerMode = schedulerMode;
else
    statusSchedulerMode = 0;
end

statusSafetyValid = double( ...
    isfinite(safetyValid) && ...
    safetyValid > 0.5);

statusControllerEnableSafe = double( ...
    isfinite(controllerEnableSafe) && ...
    controllerEnableSafe > 0.5);

%% 固定顺序状态数组
controllerStatus = [
    statusInputDataValid
    statusCameraModelValid
    statusFocalLengthFresh
    statusKinematicsValid
    statusValidLeft
    statusValidRight
    statusValidStereoQualified
    statusEkfPredictionValid
    statusEkfMeasurementUpdated
    statusDepthTaskWeight
    statusSchedulerMode
    statusSafetyValid
    statusControllerEnableSafe
];

%% 最终机械臂输出许可
armCommandEnable = ...
    all(isfinite(qDot)) && ...
    statusInputDataValid > 0.5 && ...
    statusCameraModelValid > 0.5 && ...
    statusKinematicsValid > 0.5 && ...
    statusValidLeft > 0.5 && ...
    statusSafetyValid > 0.5 && ...
    statusControllerEnableSafe > 0.5;

if armCommandEnable
    jointVelocityCmd = qDot;
end

%% 最终Zoom输出许可
zoomCommandEnable = ...
    all(isfinite(fDotMm)) && ...
    statusInputDataValid > 0.5 && ...
    statusCameraModelValid > 0.5 && ...
    statusFocalLengthFresh > 0.5 && ...
    statusValidLeft > 0.5 && ...
    statusSafetyValid > 0.5 && ...
    statusControllerEnableSafe > 0.5;

if zoomCommandEnable
    focalRateCmdMmPerSec = fDotMm;
end

%% 最终有限值保护
if any(~isfinite(jointVelocityCmd))
    jointVelocityCmd = zeros(7,1);
end

if any(~isfinite(focalRateCmdMmPerSec))
    focalRateCmdMmPerSec = zeros(2,1);
end

if any(~isfinite(controllerStatus))
    controllerStatus = zeros(13,1);
end
end

== matlab function stereo_ibvs_core_backup_20260724_004703/09_Safety_Supervisor/Apply Safety and Saturation ==
  data: qDotCmd input; qDotApplied output; fDotMmLimited input; q input; focalLengthMeasuredMm input; validLeft input; focalLengthFresh input; cameraModelValid input; kinematicsValid input; JL input; controllerEnableSafe input; cfg_qDotMax input; cfg_qDotAlgorithmMax input; cfg_qMin input; cfg_qMax input; cfg_qLimitSoftMargin input; cfg_cartesianLinearSpeedMax input; cfg_focalRateGuaranteedMmPerSec input; cfg_focalRateAbsoluteMaxMmPerSec input; cfg_focalLengthWorkingMinMm input; cfg_focalLengthWorkingMaxMm input; cfg_focalLengthHardwareMinMm input; cfg_focalLengthHardwareMaxMm input; cfg_Ts input; cfg_numericalEpsilon input; cfg_armControlCalibrationReady input; cfg_zoomControlCalibrationReady input; cfg_armControlEnable input; cfg_zoomControlEnable input; fDotMmApplied output; qSaturationFlag output; focalRateSaturationFlag output; jointVelocitySaturationFlag output; jointVelocitySaturationAny output; jointLimitWarning output; cartesianSpeed output; cartesianSpeedScale output; cartesianSpeedSaturationFlag output; focalLengthCommandMm output; focalRateUsageGuaranteed output; focalRateUsageHard output; focalRateHardViolation output; safetyValid output
function [ ...
    qDotApplied, ...
    fDotMmApplied, ...
    qSaturationFlag, ...
    focalRateSaturationFlag, ...
    jointVelocitySaturationFlag, ...
    jointVelocitySaturationAny, ...
    jointLimitWarning, ...
    cartesianSpeed, ...
    cartesianSpeedScale, ...
    cartesianSpeedSaturationFlag, ...
    focalLengthCommandMm, ...
    focalRateUsageGuaranteed, ...
    focalRateUsageHard, ...
    focalRateHardViolation, ...
    safetyValid] = fcn( ...
    qDotCmd, ...
    fDotMmLimited, ...
    q, ...
    focalLengthMeasuredMm, ...
    validLeft, ...
    focalLengthFresh, ...
    cameraModelValid, ...
    kinematicsValid, ...
    JL, ...
    controllerEnableSafe, ...
    cfg_qDotMax, ...
    cfg_qDotAlgorithmMax, ...
    cfg_qMin, ...
    cfg_qMax, ...
    cfg_qLimitSoftMargin, ...
    cfg_cartesianLinearSpeedMax, ...
    cfg_focalRateGuaranteedMmPerSec, ...
    cfg_focalRateAbsoluteMaxMmPerSec, ...
    cfg_focalLengthWorkingMinMm, ...
    cfg_focalLengthWorkingMaxMm, ...
    cfg_focalLengthHardwareMinMm, ...
    cfg_focalLengthHardwareMaxMm, ...
    cfg_Ts, ...
    cfg_numericalEpsilon, ...
    cfg_armControlCalibrationReady, ...
    cfg_zoomControlCalibrationReady, ...
    cfg_armControlEnable, ...
    cfg_zoomControlEnable)
%#codegen
% V2 Safety and Saturation
% JL顺序：[linear velocity; angular velocity]

%% 固定尺寸输出
qDotApplied = zeros(7,1);
fDotMmApplied = zeros(2,1);

qSaturationFlag = 0;
focalRateSaturationFlag = 0;

jointVelocitySaturationFlag = zeros(7,1);
jointVelocitySaturationAny = 0;
jointLimitWarning = zeros(7,1);

cartesianSpeed = 0;
cartesianSpeedScale = 1;
cartesianSpeedSaturationFlag = 0;

focalLengthCommandMm = zeros(2,1);
focalRateUsageGuaranteed = zeros(2,1);
focalRateUsageHard = zeros(2,1);
focalRateHardViolation = zeros(2,1);

safetyValid = 0;

%% 固定尺寸输入
qDotRequested = reshape(qDotCmd,7,1);
fDotRequested = reshape(fDotMmLimited,2,1);
qMeasured = reshape(q,7,1);
focalMeasured = reshape(focalLengthMeasuredMm,2,1);

%% 参数检查
tol = max(cfg_numericalEpsilon,1e-12);

inputFinite = ...
    all(isfinite(qDotRequested)) && ...
    all(isfinite(fDotRequested)) && ...
    all(isfinite(qMeasured)) && ...
    all(isfinite(focalMeasured)) && ...
    all(isfinite(JL(:))) && ...
    isfinite(validLeft) && ...
    isfinite(focalLengthFresh) && ...
    isfinite(cameraModelValid) && ...
    isfinite(kinematicsValid) && ...
    isfinite(controllerEnableSafe);

parameterFinite = ...
    all(isfinite(cfg_qDotMax)) && ...
    all(isfinite(cfg_qDotAlgorithmMax)) && ...
    all(isfinite(cfg_qMin)) && ...
    all(isfinite(cfg_qMax)) && ...
    isfinite(cfg_qLimitSoftMargin) && ...
    isfinite(cfg_cartesianLinearSpeedMax) && ...
    isfinite(cfg_focalRateGuaranteedMmPerSec) && ...
    isfinite(cfg_focalRateAbsoluteMaxMmPerSec) && ...
    all(isfinite(cfg_focalLengthWorkingMinMm)) && ...
    all(isfinite(cfg_focalLengthWorkingMaxMm)) && ...
    all(isfinite(cfg_focalLengthHardwareMinMm)) && ...
    all(isfinite(cfg_focalLengthHardwareMaxMm)) && ...
    isfinite(cfg_Ts) && ...
    isfinite(cfg_numericalEpsilon) && ...
    isfinite(cfg_armControlCalibrationReady) && ...
    isfinite(cfg_zoomControlCalibrationReady) && ...
    isfinite(cfg_armControlEnable) && ...
    isfinite(cfg_zoomControlEnable);

parameterRangesValid = ...
    all(cfg_qDotMax >= 0) && ...
    all(cfg_qDotAlgorithmMax >= 0) && ...
    all(cfg_qMax > cfg_qMin) && ...
    cfg_qLimitSoftMargin >= 0 && ...
    all(2*cfg_qLimitSoftMargin < ...
        (cfg_qMax-cfg_qMin)) && ...
    cfg_cartesianLinearSpeedMax > 0 && ...
    cfg_focalRateGuaranteedMmPerSec > 0 && ...
    cfg_focalRateAbsoluteMaxMmPerSec >= ...
        cfg_focalRateGuaranteedMmPerSec && ...
    all(cfg_focalLengthHardwareMaxMm > ...
        cfg_focalLengthHardwareMinMm) && ...
    all(cfg_focalLengthWorkingMinMm >= ...
        cfg_focalLengthHardwareMinMm) && ...
    all(cfg_focalLengthWorkingMaxMm <= ...
        cfg_focalLengthHardwareMaxMm) && ...
    all(cfg_focalLengthWorkingMaxMm > ...
        cfg_focalLengthWorkingMinMm) && ...
    cfg_Ts > 0;

if ~(inputFinite && parameterFinite && parameterRangesValid)
    qSaturationFlag = 1;
    focalRateSaturationFlag = 1;
    jointVelocitySaturationFlag = ones(7,1);
    jointVelocitySaturationAny = 1;
    cartesianSpeedScale = 0;
    return;
end

safetyValid = 1;

%% 当前焦距
if cameraModelValid > 0.5
    focalLengthCommandMm = focalMeasured;
end

%% 关节限位诊断
for i = 1:7
    nearLowerLimit = ...
        qMeasured(i) <= ...
        cfg_qMin(i)+cfg_qLimitSoftMargin;

    nearUpperLimit = ...
        qMeasured(i) >= ...
        cfg_qMax(i)-cfg_qLimitSoftMargin;

    outsideLowerLimit = ...
        qMeasured(i) <= cfg_qMin(i);

    outsideUpperLimit = ...
        qMeasured(i) >= cfg_qMax(i);

    jointLimitWarning(i) = double( ...
        nearLowerLimit || ...
        nearUpperLimit || ...
        outsideLowerLimit || ...
        outsideUpperLimit);
end

%% 控制许可
armPermission = ...
    controllerEnableSafe > 0.5 && ...
    cfg_armControlEnable > 0.5 && ...
    cfg_armControlCalibrationReady > 0.5 && ...
    validLeft > 0.5 && ...
    cameraModelValid > 0.5 && ...
    kinematicsValid > 0.5;

zoomPermission = ...
    controllerEnableSafe > 0.5 && ...
    cfg_zoomControlEnable > 0.5 && ...
    cfg_zoomControlCalibrationReady > 0.5 && ...
    validLeft > 0.5 && ...
    cameraModelValid > 0.5 && ...
    focalLengthFresh > 0.5;

%% 关节速度限制
if armPermission

    qDotLimit = min( ...
        abs(cfg_qDotMax), ...
        abs(cfg_qDotAlgorithmMax));

    qCandidate = min( ...
        max(qDotRequested,-qDotLimit), ...
        qDotLimit);

    for i = 1:7

        nearLowerLimit = ...
            qMeasured(i) <= ...
            cfg_qMin(i)+cfg_qLimitSoftMargin;

        nearUpperLimit = ...
            qMeasured(i) >= ...
            cfg_qMax(i)-cfg_qLimitSoftMargin;

        if nearLowerLimit && qCandidate(i) < 0
            qCandidate(i) = 0;
        end

        if nearUpperLimit && qCandidate(i) > 0
            qCandidate(i) = 0;
        end
    end

    %% 笛卡尔线速度限制
    cameraTwistCandidate = JL*qCandidate;
    cartesianSpeedCandidate = ...
        norm(cameraTwistCandidate(1:3));

    if ~isfinite(cartesianSpeedCandidate)

        qCandidate = zeros(7,1);
        cartesianSpeedScale = 0;
        cartesianSpeedSaturationFlag = 1;
        safetyValid = 0;

    elseif cartesianSpeedCandidate > ...
            cfg_cartesianLinearSpeedMax

        cartesianSpeedScale = ...
            cfg_cartesianLinearSpeedMax / ...
            max(cartesianSpeedCandidate,tol);

        qCandidate = ...
            cartesianSpeedScale*qCandidate;

        cartesianSpeedSaturationFlag = 1;
    end

    qDotApplied = min( ...
        max(qCandidate,-qDotLimit), ...
        qDotLimit);

    finalCameraTwist = JL*qDotApplied;
    cartesianSpeed = norm(finalCameraTwist(1:3));
end

%% Zoom硬限速违规诊断
focalRateHardViolation = double( ...
    abs(fDotRequested) > ...
    cfg_focalRateAbsoluteMaxMmPerSec);

%% Zoom焦距速度限制
if zoomPermission

    fCandidate = min( ...
        max(fDotRequested, ...
            -cfg_focalRateAbsoluteMaxMmPerSec), ...
        cfg_focalRateAbsoluteMaxMmPerSec);

    for i = 1:2

        focalCurrent = focalMeasured(i);

        workingMin = ...
            cfg_focalLengthWorkingMinMm(i);
        workingMax = ...
            cfg_focalLengthWorkingMaxMm(i);

        hardwareMin = ...
            cfg_focalLengthHardwareMinMm(i);
        hardwareMax = ...
            cfg_focalLengthHardwareMaxMm(i);

        %% 禁止继续远离工作范围
        if focalCurrent <= workingMin && ...
                fCandidate(i) < 0
            fCandidate(i) = 0;
        end

        if focalCurrent >= workingMax && ...
                fCandidate(i) > 0
            fCandidate(i) = 0;
        end

        %% 下一周期工作范围预测
        nextFocalLength = ...
            focalCurrent + ...
            cfg_Ts*fCandidate(i);

        if focalCurrent >= workingMin && ...
                nextFocalLength < workingMin

            fCandidate(i) = ...
                (workingMin-focalCurrent)/cfg_Ts;

        elseif focalCurrent <= workingMax && ...
                nextFocalLength > workingMax

            fCandidate(i) = ...
                (workingMax-focalCurrent)/cfg_Ts;
        end

        %% 硬件范围最终保护
        nextFocalLength = ...
            focalCurrent + ...
            cfg_Ts*fCandidate(i);

        if nextFocalLength < hardwareMin

            fCandidate(i) = ...
                (hardwareMin-focalCurrent)/cfg_Ts;

        elseif nextFocalLength > hardwareMax

            fCandidate(i) = ...
                (hardwareMax-focalCurrent)/cfg_Ts;
        end
    end

    fDotMmApplied = min( ...
        max(fCandidate, ...
            -cfg_focalRateAbsoluteMaxMmPerSec), ...
        cfg_focalRateAbsoluteMaxMmPerSec);
end

%% 最终有限值保护
if any(~isfinite(qDotApplied)) || ...
        ~isfinite(cartesianSpeed) || ...
        ~isfinite(cartesianSpeedScale)

    qDotApplied = zeros(7,1);
    cartesianSpeed = 0;
    cartesianSpeedScale = 0;
    cartesianSpeedSaturationFlag = 1;
    safetyValid = 0;
end

if any(~isfinite(fDotMmApplied))
    fDotMmApplied = zeros(2,1);
    safetyValid = 0;
end

%% 饱和诊断
jointVelocitySaturationFlag = double( ...
    abs(qDotApplied-qDotRequested) > tol);

jointVelocitySaturationAny = double( ...
    any(jointVelocitySaturationFlag > 0.5));

qSaturationFlag = ...
    jointVelocitySaturationAny;

focalRateSaturationFlag = double( ...
    any(abs(fDotMmApplied-fDotRequested) > tol));

%% Zoom使用率
focalRateUsageGuaranteed = ...
    abs(fDotMmApplied) / ...
    cfg_focalRateGuaranteedMmPerSec;

focalRateUsageHard = ...
    abs(fDotMmApplied) / ...
    cfg_focalRateAbsoluteMaxMmPerSec;

%% 下一周期焦距命令
if cameraModelValid > 0.5

    focalLengthCommandMm = min( ...
        max( ...
            focalMeasured + ...
            cfg_Ts*fDotMmApplied, ...
            cfg_focalLengthHardwareMinMm), ...
        cfg_focalLengthHardwareMaxMm);

else
    focalLengthCommandMm = zeros(2,1);
end

%% 最终输出检查
if any(~isfinite(focalLengthCommandMm)) || ...
        any(~isfinite(focalRateUsageGuaranteed)) || ...
        any(~isfinite(focalRateUsageHard))

    fDotMmApplied = zeros(2,1);
    focalLengthCommandMm = zeros(2,1);
    focalRateUsageGuaranteed = zeros(2,1);
    focalRateUsageHard = zeros(2,1);
    safetyValid = 0;
end
end

== matlab function stereo_ibvs_core_backup_20260724_004703/06_Estimated_Rho_Dynamics/Estimate Rho Dynamics ==
  data: normalizedFeatureMeasured input; rhoDotHat output; rhoHatSafe input; vHatCL input; vHatCR input; JL input; JR input; qDotAppliedDelayed input; cfg_numericalEpsilon input; rhoDynamicsValid output
function [rhoDotHat, rhoDynamicsValid] = fcn( ...
    normalizedFeatureMeasured, ...
    rhoHatSafe, ...
    vHatCL, ...
    vHatCR, ...
    JL, ...
    JR, ...
    qDotAppliedDelayed, cfg_numericalEpsilon)
%#codegen
% V2 Estimated Rho Dynamics
%
% 输入尺寸：
% normalizedFeatureMeasured : 4×1 [xL;yL;xR;yR]
% rhoHatSafe                : 1×1
% vHatCL                    : 3×1
% vHatCR                    : 3×1
% JL                        : 6×7
% JR                        : 6×7
% qDotAppliedDelayed        : 7×1
%
% 输出：
% rhoDotHat                 : 2×1
% rhoDynamicsValid          : 1×1

%% 固定尺寸输出
rhoDotHat = zeros(2,1);
rhoDynamicsValid = false;

features = reshape(normalizedFeatureMeasured,4,1);
velocityCL = reshape(vHatCL,3,1);
velocityCR = reshape(vHatCR,3,1);
qDotDelayed = reshape(qDotAppliedDelayed,7,1);

%% 输入有效性
inputValid = ...
    all(isfinite(features)) && ...
    isfinite(rhoHatSafe) && ...
    all(isfinite(velocityCL)) && ...
    all(isfinite(velocityCR)) && ...
    all(isfinite(JL(:))) && ...
    all(isfinite(JR(:))) && ...
    all(isfinite(qDotDelayed)) && ...
    isfinite(cfg_numericalEpsilon) && ...
    cfg_numericalEpsilon > 0 && ...
    rhoHatSafe > cfg_numericalEpsilon;

if ~inputValid
    return;
end

rho = max(rhoHatSafe, cfg_numericalEpsilon);

%% 左相机
xL = features(1);
yL = features(2);

LrhoL = [
    0, 0, rho*rho, ...
    rho*yL, -rho*xL, 0
];

Hrho = [0, 0, -rho*rho];

cameraVelocityLeft = JL * qDotDelayed;

rhoDotHat(1) = ...
    LrhoL * cameraVelocityLeft + ...
    Hrho * velocityCL;

%% 右相机
xR = features(3);
yR = features(4);

LrhoR = [
    0, 0, rho*rho, ...
    rho*yR, -rho*xR, 0
];

cameraVelocityRight = JR * qDotDelayed;

rhoDotHat(2) = ...
    LrhoR * cameraVelocityRight + ...
    Hrho * velocityCR;

%% 最终数值保护
if all(isfinite(rhoDotHat))
    rhoDynamicsValid = true;
else
    rhoDotHat = zeros(2,1);
    rhoDynamicsValid = false;
end
end
